simulink subsystem "Intersection_Long_Lat_Generator_Sub"  (R2024b)
settings: Solver=VariableStepAuto  StartTime=0.0  StopTime=10.0  RelTol=1e-3
libraries: simulink x1
settings Model: Creator=nelsenyoung  LastModifiedBy=nelsenyoung

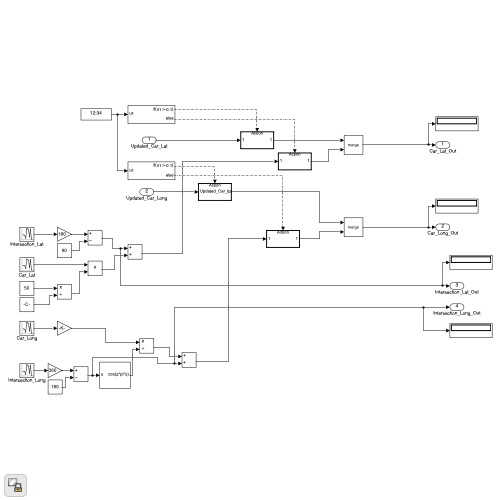
[thumbnail: Simulink's stored preview of the top-level diagram]
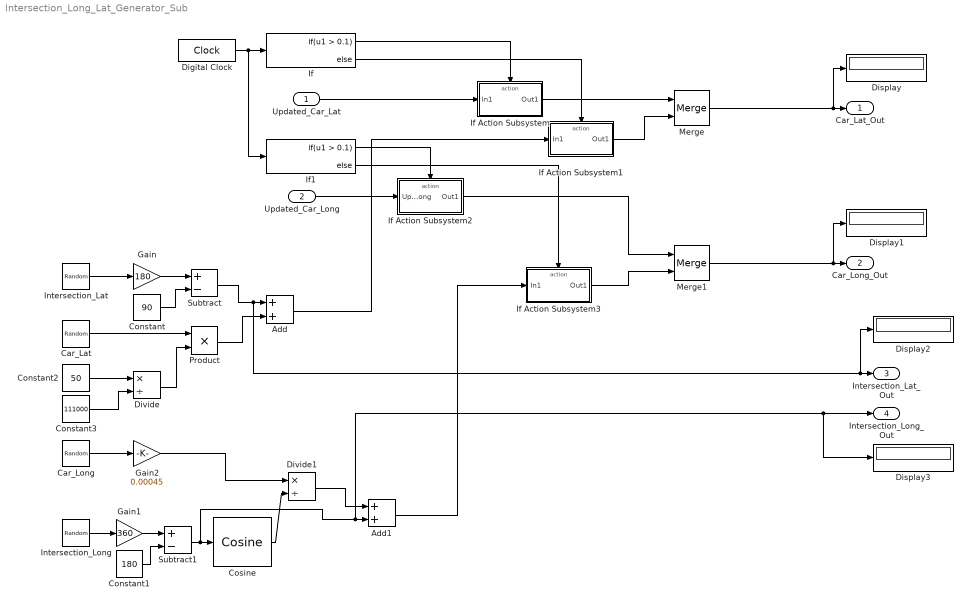
== system Intersection_Long_Lat_Generator_Sub ==
  Updated_Car_Lat : Inport
  Updated_Car_Long : Inport  Port=2
  Add : Sum
  Add1 : Sum
  Car_Lat : RandomNumber  SampleTime=10000
  Car_Long : RandomNumber  SampleTime=10000
  Constant : Constant  Value=90
  Constant1 : Constant  Value=180
  Constant2 : Constant  Value=50
  Constant3 : Constant  Value=111000
  Cosine : simulink/Lookup Tables/Cosine  Formula=cos(2*pi*u)  NumDataPoints=(2^5)+1  OutputWordLength=16  InternalRulePriority=Speed
  Digital Clock : DigitalClock  SampleTime=0.1
  Display{,1..3} (4 alike) : Display
  Divide : Product  Inputs=*/
  Divide1 : Product  Inputs=*/
  Gain : Gain  Gain=180
  Gain1 : Gain  Gain=360
  Gain2 : Gain  Gain=0.00045
  If : If  IfExpression=u1 > 0.1
  If Action Subsystem : Subsystem  TreatAsAtomicUnit=on
  If Action Subsystem1 : Subsystem  TreatAsAtomicUnit=on
  If Action Subsystem2 : Subsystem  TreatAsAtomicUnit=on
  If Action Subsystem3 : Subsystem  TreatAsAtomicUnit=on
  If1 : If  IfExpression=u1 > 0.1
  Intersection_Lat : RandomNumber  SampleTime=10000
  Intersection_Long : RandomNumber  SampleTime=10000
  Merge : Merge
  Merge1 : Merge
  Product : Product
  Subtract : Sum  Inputs=+-
  Subtract1 : Sum  Inputs=+-
  Car_Lat_Out : Outport
  Car_Long_Out : Outport  Port=2
  Intersection_Lat_Out : Outport  Port=3
  Intersection_Long_Out : Outport  Port=4
  wires:
  If Action Subsystem2/1(Out1) -> Merge1/1
  Car_Long/1 -> Gain2/1
  If1/2 -> If Action Subsystem3/Action
  Divide1/1 -> Add1/1
  Merge1/1 -> Car_Long_Out/1, Display1/1
  Intersection_Long/1 -> Gain1/1
  Cosine/1 -> Divide1/2
  Updated_Car_Lat/1 -> If Action Subsystem/1(In1)
  Constant/1 -> Subtract/2
  If/1 -> If Action Subsystem/Action
  Divide/1 -> Product/2
  Constant2/1 -> Divide/1
  Add1/1 -> If Action Subsystem3/1(In1)
  If Action Subsystem3/1(Out1) -> Merge1/2
  Digital Clock/1 -> If/1, If1/1
  Intersection_Lat/1 -> Gain/1
  Gain/1 -> Subtract/1
  Add/1 -> If Action Subsystem1/1(In1)
  If1/1 -> If Action Subsystem2/Action
  Subtract1/1 -> Cosine/1, Add1/2, Display3/1, Intersection_Long_Out/1
  Gain1/1 -> Subtract1/1
  If Action Subsystem/1(Out1) -> Merge/1
  Car_Lat/1 -> Product/1
  Constant1/1 -> Subtract1/2
  Subtract/1 -> Add/1, Intersection_Lat_Out/1, Display2/1
  Gain2/1 -> Divide1/1
  If/2 -> If Action Subsystem1/Action
  If Action Subsystem1/1(Out1) -> Merge/2
  Constant3/1 -> Divide/2
  Merge/1 -> Car_Lat_Out/1, Display/1
  Product/1 -> Add/2
  Updated_Car_Long/1 -> If Action Subsystem2/1(Updated_Car_Long)

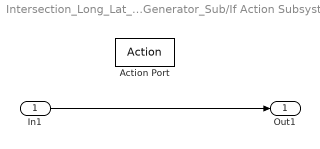
== system Intersection_Long_Lat_Generator_Sub/If Action Subsystem ==
  In1 : Inport
  Action Port : ActionPort
  Out1 : Outport
  wires:
  In1/1 -> Out1/1

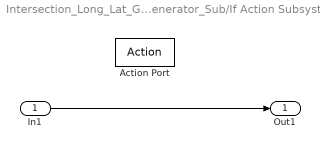
== system Intersection_Long_Lat_Generator_Sub/If Action Subsystem1 ==
  In1 : Inport
  Action Port : ActionPort
  Out1 : Outport
  wires:
  In1/1 -> Out1/1

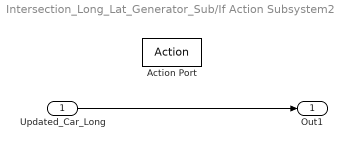
== system Intersection_Long_Lat_Generator_Sub/If Action Subsystem2 ==
  Updated_Car_Long : Inport
  Action Port : ActionPort
  Out1 : Outport
  wires:
  Updated_Car_Long/1 -> Out1/1

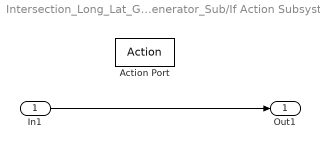
== system Intersection_Long_Lat_Generator_Sub/If Action Subsystem3 ==
  In1 : Inport
  Action Port : ActionPort
  Out1 : Outport
  wires:
  In1/1 -> Out1/1
